simulink model "FMLibrary_v2_progress"  (R2016b)
settings: Solver=VariableStepAuto  StartTime=0.0  StopTime=10.0  RelTol=1e-3
undefined symbols (not defined in the file or in its folder): Lb, Lf, Lu, RobotStruct, sampleTime
libraries: simulink x24, FM_Library x10, VariousBlocksLibrary x10, FMLibrary_v2 x2, simulink_extras x2
(part 3 of 3)

== matlab function FMLibrary_v2_progress/Robot1/Controller/run1/reference ==
  data: t input; p output; v output; a output; T input; n input; hstart input; hend input; wstart input; wend input
function [p,v,a] = fcn(t,T,n,hstart,hend,wstart,wend)
%#codegen

% T = 80;
% hstart = 0.02;
% hend = 0.02;
% n = 5;
% wstart = 0.5;%0.2*2*pi;
% wend = 0.5;%0.2*2*pi;

p = func_p_hypothrochoid(t,T,n,hstart,hend,wstart,wend);
v = func_v_hypothrochoid(t,T,n,hstart,hend,wstart,wend);
a = func_a_hypothrochoid(t,T,n,hstart,hend,wstart,wend);

== matlab function FMLibrary_v2_progress/Robot1/DataToEtherCAT_FM/ToActuator1/DriveEnableLogic/64_DriveError/CountHowLongEnableWasTrue ==
  data: u input; y output
function y = fcn(u)
%#codegen
%
% This block counts how many samples the input has been on (true). As soon
% as the input goes false, the counter is reset.
persistent onCounter;

if isempty(onCounter)
    onCounter = 0;
end;

if u == 1
    onCounter = onCounter + 1;
else
    % u == 0
    onCounter = 0;
end;
y = onCounter;

== matlab function FMLibrary_v2_progress/Robot1/DataFromEtherCAT_FM/Calculate//Arrange Joint and Op Space/forward kinematics/Je ==
  data: q input; Je output size=[2 2]; Lf parameter; Lu parameter; Lb parameter
function Je = Je( q, Lf, Lu, Lb)
%#codegen

% Calculate the Jacobian for this particular device configuration.
% Note that the function func_eq_Je needs to be in the libraries/kinematis_functions folder

% jacobians
Je = func_eq_Je(q(1),q(2),Lf,Lu,Lb);

== matlab function FMLibrary_v2_progress/Robot1/DataFromEtherCAT_FM/Calculate//Arrange Joint and Op Space/forward kinematics/Jedot ==
  data: q input; qdot input; Jedot output size=[2 2]; Lf parameter; Lu parameter; Lb parameter
function Jedot = Jedot( q, qdot, Lf, Lu, Lb)
%#codegen

% Calculate the time derivative of the Jacobian for this particular device configuration.
% Note that the function func_eq_Je needs to be in the libraries/kinematis_functions folder


% jacobians
Jedot = func_eq_Jedot(q(1),q(2),qdot(1),qdot(2),Lf,Lu,Lb);

== matlab function FMLibrary_v2_progress/Robot1/DataFromEtherCAT_FM/FTSensor_K6D27/CorrectOffset ==
  data: u_in input; u_out output; reset input; corrected output
function [u_out,corrected] = CorrectOffset(u_in,reset)
%#codegen

persistent data_ offset_ counter_ corrected_;
N = 1000;

% initialize
if isempty(data_)
    data_ = zeros(size(u_in,1), N);
    offset_ = zeros(size(u_in));
    counter_ = 1;
    corrected_ = 0;
end

if (counter_ <= N)
    data_(:,counter_) = u_in;
end

counter_ = counter_ + 1;
if reset
    counter_ = 1;
end

% calculate mean
if counter_ == N
    corrected_ = 1;
    offset_ = mean(data_,2);
end

corrected = corrected_;
u_out = u_in - offset_;

== matlab function FMLibrary_v2_progress/Robot1/DataFromEtherCAT_FM/FromActuator1/CheckOperationEnabled ==
  data: u input; y output
function y = fcn(u)
%#codegen

mask  = bin2dec('0000000001101111');
match = bin2dec('0000000000100111');

masked = bitand(u,mask);
if masked==match
    y=1;
else
    y=0;
end;

== matlab function FMLibrary_v2_progress/Robot1/DataFromEtherCAT_FM/Calculate//Arrange Joint and Op Space/IK all joints ==
  data: x input; q_all output; Lf parameter; Lu parameter; Lb parameter
function q_all = IK_all(x,Lf,Lu,Lb)
%#codegen

if (x(2) >= 0.07)
    q_all = func_eqs_IK_all(x(1),x(2),Lf,Lu,Lb);
else
    x = [0;0.07];
    q_all = func_eqs_IK_all(x(1),x(2),Lf,Lu,Lb);
end

== matlab function FMLibrary_v2_progress/Robot1/DataFromEtherCAT_FM/Calculate//Arrange Joint and Op Space/forward kinematics/calculate xddot ==
  data: qddot input; qdot input size=[2 1]; J input; xddot output size=[2 1]; Jdot input
function xddot = calc_xddot(qddot, qdot, J, Jdot)
%#codegen

xddot = J*qddot + Jdot*qdot;

== matlab function FMLibrary_v2_progress/Robot1/Controller/inverse kinematics ==
  data: x input; xdot input; xddot input; q output size=[2 1]; Lf parameter; Lu parameter; Lb parameter; qdot output; qddot output
function [q,qdot,qddot] = IK(x,xdot,xddot,Lf,Lu,Lb)
%#codegen

% inverse dynamics
q = func_eq_IK(x(1),x(2),Lf,Lu,Lb);

% jacobians
Je = func_eq_Je(q(1),q(2),Lf,Lu,Lb);

% calculate qdot
qdot = Je\xdot;

% calculate qddot
Jedot = func_eq_Jedot(q(1),q(2),qdot(1),qdot(2),Lf,Lu,Lb);
qddot = Je\(xddot-Jedot*qdot);

== matlab function FMLibrary_v2_progress/Robot1/DataToEtherCAT_FM/ToActuator1/DriveEnableLogic/CreateSingleErrorValue/MATLAB Function ==
  data: errors input; out output
function out = errorToPowerOf2(errors)
%#codegen

% if size(errors,1) > size(errors,2)
%     errors = errors.';
% end
out = sum(errors.*(2.^(0:(length(errors)-1)).'));

== matlab function FMLibrary_v2_progress/Robot1/DataToEtherCAT_FM/ToActuator1/DriveEnableLogic/enableDrive (CoE) ==
  data: ControlWord output; enable input; TimePerState_ms input
function ControlWord = enabledrive(enable, TimePerState_ms)
%#codegen
%
% Input arguments:
% enable:
%   0: Disable drive
%   Any non-zero: enable drive.
% TimePerState_ms:
%   A four-element array containing the time in ms for each state (states
%   are: 0, 128, 6, 7. The final state, 15, is kept until drive needs to be
%   disabled again.
%
% Changing enable forces the initialize-sequence to run
persistent previousEnable;
persistent counter;
if isempty(previousEnable)
    previousEnable = enable; % No enabling of the drive at startup
    counter = 1e6;
end;

if enable~=previousEnable
    counter = 0;
end;
previousEnable = enable;

TimePerState_cum = cumsum(TimePerState_ms);

if enable~=0
    counter = counter+1;
    if counter < TimePerState_cum(1);
        ControlWord_ = 0;
    elseif counter < TimePerState_cum(2);
        ControlWord_ = 128;
    elseif counter < TimePerState_cum(3);
        ControlWord_ = 6;
    elseif counter < TimePerState_cum(4);
        ControlWord_ = 7;
    else
        ControlWord_ = 15;
    end
else
    ControlWord_ = 6;
end

ControlWord = uint16(ControlWord_);

== matlab function FMLibrary_v2_progress/Robot1/DataToEtherCAT_FM/ToActuator1/EncodeDesiredTorque ==
  data: MotorTorque_Des_IU output int16; JointTorque_Des_Nm input; transmissionRatio parameter; motorTorqueConstant parameter; drivePeakCurrent parameter
function MotorTorque_Des_IU = EncodeDesiredTorque(JointTorque_Des_Nm, transmissionRatio, motorTorqueConstant, drivePeakCurrent)
%#codegen
% Calculate the target torque in incremental units for a desired joint
% torque.

% compute torque at motor (negate because sign change due to transmission)
torque_motor = JointTorque_Des_Nm / transmissionRatio; 

% desired current (i_des) = torque_motor / kt (torque constant)
i_des = torque_motor / motorTorqueConstant;

% calculate the target torque in incremental units [IU], see CoE manual
% Technosoftmotion
MotorTorque_Des_IU = int16( 65520*i_des / (2*drivePeakCurrent) );

== matlab function FMLibrary_v2_progress/Robot1/DataToEtherCAT_FM/ToActuator/DriveEnableLogic/64_DriveError/CountHowLongEnableWasTrue ==
  data: u input; y output
function y = fcn(u)
%#codegen
%
% This block counts how many samples the input has been on (true). As soon
% as the input goes false, the counter is reset.
persistent onCounter;

if isempty(onCounter)
    onCounter = 0;
end;

if u == 1
    onCounter = onCounter + 1;
else
    % u == 0
    onCounter = 0;
end;
y = onCounter;

== matlab function FMLibrary_v2_progress/Robot1/DataFromEtherCAT_FM/FromActuator1/DecodeActualTorque ==
  data: JointTorque_Act_Nm output; MotorCurrent_Act_IU input int16; transmissionRatio parameter; drivePeakCurrent parameter; motorTorqueConstant parameter
function JointTorque_Act_Nm = DecodeActualTorque(MotorCurrent_Act_IU, transmissionRatio, drivePeakCurrent, motorTorqueConstant)
%#codegen
%

% convert incremental units to motor torque value. See the technosoft CoE
% manual for the decoding
torquemotor_act = motorTorqueConstant * (double(MotorCurrent_Act_IU)*2*drivePeakCurrent / 65520);

% motor torque to joint torque (transmission). Negate due to sign change
% due to transmission.
JointTorque_Act_Nm = torquemotor_act * transmissionRatio;

== matlab function FMLibrary_v2_progress/Robot1/DataFromEtherCAT_FM/FromActuator1/DecodeEncoder_AbsEnc ==
  data: Encoder_counts input; EncoderCounts_rev parameter; EncoderPosition_rad output
function EncoderPosition_rad = ...
    DecodeEncoder(Encoder_counts, EncoderCounts_rev)
%#codegen

% This block decodes the motor encoder counts to the motor angle

EncoderPosition_rad = (double(Encoder_counts) / EncoderCounts_rev * 2 * pi);

== matlab function FMLibrary_v2_progress/Robot1/DataFromEtherCAT_FM/FromActuator1/DecodeEncoder_IncEnc ==
  data: Encoder_counts input; EncoderCounts_rev parameter; EncoderPosition_rad output
function EncoderPosition_rad = ...
    DecodeEncoder(Encoder_counts, EncoderCounts_rev)
%#codegen

% This block decodes the motor encoder counts to the motor angle

EncoderPosition_rad = (double(Encoder_counts) / EncoderCounts_rev * 2 * pi);

== matlab function FMLibrary_v2_progress/Robot1/DataFromEtherCAT_FM/FromActuator1/CalibrateAbsEncoder ==
  data: encoderPosition input; JointPosition_AbsEnc_rad output; offset input
function JointPosition_AbsEnc_rad = CalibrateAbsoluteEncoder(encoderPosition, offset)
%#codegen

% unwrap encoder angle (in case the encoder goes through 0
encoderPosition = unwrap(encoderPosition);

% remove offset
JointPosition_AbsEnc_rad = encoderPosition - offset;

% since the absolute encoder is mounted upside-down, negate the
% jointposition angle
JointPosition_AbsEnc_rad = -JointPosition_AbsEnc_rad;

== matlab function FMLibrary_v2_progress/Robot1/DataToEtherCAT_FM/ToActuator/DriveEnableLogic/CreateSingleErrorValue/MATLAB Function ==
  data: errors input; out output
function out = errorToPowerOf2(errors)
%#codegen

% if size(errors,1) > size(errors,2)
%     errors = errors.';
% end
out = sum(errors.*(2.^(0:(length(errors)-1)).'));

== matlab function FMLibrary_v2_progress/Robot1/DataToEtherCAT_FM/ToActuator/DriveEnableLogic/enableDrive (CoE) ==
  data: ControlWord output; enable input; TimePerState_ms input
function ControlWord = enabledrive(enable, TimePerState_ms)
%#codegen
%
% Input arguments:
% enable:
%   0: Disable drive
%   Any non-zero: enable drive.
% TimePerState_ms:
%   A four-element array containing the time in ms for each state (states
%   are: 0, 128, 6, 7. The final state, 15, is kept until drive needs to be
%   disabled again.
%
% Changing enable forces the initialize-sequence to run
persistent previousEnable;
persistent counter;
if isempty(previousEnable)
    previousEnable = enable; % No enabling of the drive at startup
    counter = 1e6;
end;

if enable~=previousEnable
    counter = 0;
end;
previousEnable = enable;

TimePerState_cum = cumsum(TimePerState_ms);

if enable~=0
    counter = counter+1;
    if counter < TimePerState_cum(1);
        ControlWord_ = 0;
    elseif counter < TimePerState_cum(2);
        ControlWord_ = 128;
    elseif counter < TimePerState_cum(3);
        ControlWord_ = 6;
    elseif counter < TimePerState_cum(4);
        ControlWord_ = 7;
    else
        ControlWord_ = 15;
    end
else
    ControlWord_ = 6;
end

ControlWord = uint16(ControlWord_);

== matlab function FMLibrary_v2_progress/Robot1/DataToEtherCAT_FM/ToActuator/EncodeDesiredTorque ==
  data: MotorTorque_Des_IU output int16; JointTorque_Des_Nm input; transmissionRatio parameter; motorTorqueConstant parameter; drivePeakCurrent parameter
function MotorTorque_Des_IU = EncodeDesiredTorque(JointTorque_Des_Nm, transmissionRatio, motorTorqueConstant, drivePeakCurrent)
%#codegen
% Calculate the target torque in incremental units for a desired joint
% torque.

% compute torque at motor (negate because sign change due to transmission)
torque_motor = JointTorque_Des_Nm / transmissionRatio; 

% desired current (i_des) = torque_motor / kt (torque constant)
i_des = torque_motor / motorTorqueConstant;

% calculate the target torque in incremental units [IU], see CoE manual
% Technosoftmotion
MotorTorque_Des_IU = int16( 65520*i_des / (2*drivePeakCurrent) );

== matlab function FMLibrary_v2_progress/Robot1/DataFromEtherCAT_FM/FTSensor_K6D27/SensorOutputToForce1 ==
  data: FT output; u input; calibrationMatrix input; offset input
function FT = VtoF(u, calibrationMatrix, offset)
%#codegen

% ME supplies a zero offset voltages. If 
if ~isempty(offset)
    u = u + offset;
end

% Calculate forces and torques (in sensor space)
FT = calibrationMatrix*u;

== matlab function FMLibrary_v2_progress/Robot1/DataFromEtherCAT_FM/FTSensor_K6D27/SensorToOperationalSpace ==
  data: q_all input; Fs input; FTOpSpace output
function FTOpSpace = ForceSensorToOperationalSpace(q_all,Fs)
%#codegen

% select correct angles. Note! During assembly we weren't very consistent
% to which forearm the sensor is fixed. For FM1 (green), the sensor is
% attached to arm 2, hence the rotation matrics are made using angles
% theta1 and theta2
% rotation matrices (I derived them from actuator 1 to endpoint, but
% transformation is other way around (i.e. inverse). Since inverse calculation 
% could take some time, Could be done by
% negating the angles instead of inverse of matrix.
theta1 = theta_all(1);
theta2 = (pi-theta_all(2)); % pi-theta2 since theta2 is the internal angle of this joint

R = [-cos(theta1+theta2) sin(theta1+theta2);-sin(theta1+theta2) -cos(theta1+theta2)];

% transform force
FTOpSpace = R*Fs(1:2);

== matlab function FMLibrary_v2_progress/Robot1/DataToEtherCAT_FM/WorkspacePositionGuard/CheckForSingularity ==
  data: J input; kappa output
function kappa = conditionnumber(J)
%#codegen

kappa = norm(pinv(J))*norm(J);

== matlab function FMLibrary_v2_progress/Robot1/DataToEtherCAT_FM/WorkspacePositionGuard/CheckInternalAngles ==
  data: theta input; angleError output; isCalibrated input
function angleError = checkInternalErrors(theta,isCalibrated)
%#codegen

angleError = 0;

if isCalibrated
    % check whether theta2 or theta4 are smaller than 0.95*pi. If larger, throw
    % error
    if any(theta([2 4]) >= 0.95*pi)
        angleError = 1;
    end
end

== matlab function FMLibrary_v2_progress/Robot1/DataToEtherCAT_FM/WorkspacePositionGuard/CreateSingleErrorValue/MATLAB Function ==
  data: errors input; out output
function out = errorToPowerOf2(errors)
%#codegen

% if size(errors,1) > size(errors,2)
%     errors = errors.';
% end
out = sum(errors.*(2.^(0:(length(errors)-1)).'));

== matlab function FMLibrary_v2_progress/Robot1/DataToEtherCAT_FM/WorkspacePositionGuard/EndpointPositionGuard ==
  data: xe input; error output; correctState input
function error = fcn(xe, correctState)
%#codegen


error = 0;

% only check workspace boundaries after homing state is done
if ~correctState 
    return; 
end

% x0 = 0;
% y0 = 0.2354;
% a = 0.11;
% b = 0.08;

% workspace (see design document)
x0 = 0;
y0 = 0.25024;
a = 0.1746;
b = 0.13;%0.1048;

% check if endpoint is outside a predefined ellipse
x = xe(1);
y = xe(2);

% workspace is defined as an ellipse
e = (x-x0)^2 / a^2 + (y-y0)^2 / b^2;

% if is larger than 1, the endpoint is outside the workspace
if e > 1
    error = 1;
end
